simulink model "chap1_4"  (Simulink 3.00)
settings: Solver=ode45  StartTime=0.0  StopTime=5  RelTol=1e-3
libraries: simulink3 x1, simulink_extras x1

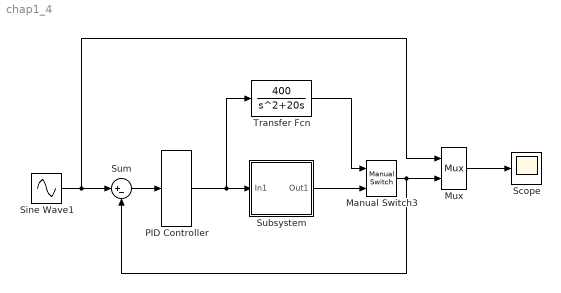
== system chap1_4 ==
  Manual Switch3 : simulink3/Nonlinear/Manual Switch  sw=0  action=0
  Mux : Mux  Inputs=2
      settings: DisplayOption=none
  PID Controller : simulink_extras/Additional Linear/PID Controller  P=10  I=0  D=1
  Scope : Scope
      settings: TimeRange=auto  YMin=-5  YMax=5  SaveToWorkspace=off  SaveName=ScopeData
  Sine Wave1 : Sin  Amplitude=0.50  Frequency=1*2*pi  Phase=0  SampleTime=0
  Subsystem : Subsystem
  Sum : Sum  Inputs=|+-  SaturateOnIntegerOverflow=on
  Transfer Fcn : TransferFcn  Numerator=[400]  Denominator=[1 20 0]
  wires:
  Sum/1 -> PID Controller/1
  Sine Wave1/1 -> Sum/1, Mux/1
  Mux/1 -> Scope/1
  Subsystem/1(Out1) -> Manual Switch3/2
  Transfer Fcn/1 -> Manual Switch3/1
  PID Controller/1 -> Subsystem/1(In1), Transfer Fcn/1
  Manual Switch3/1 -> Mux/2, Sum/2

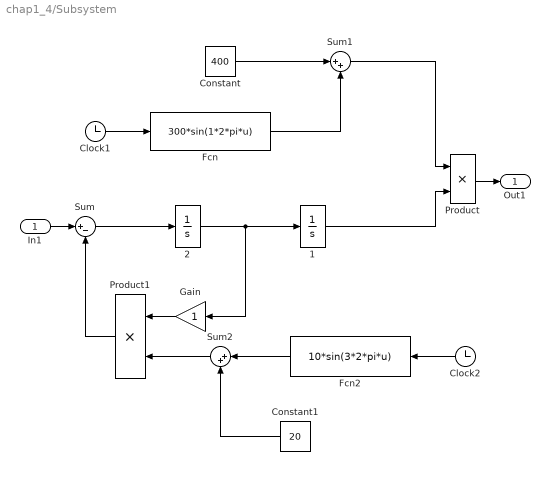
== system chap1_4/Subsystem ==
  In1 : Inport  Port=1  PortWidth=-1  SampleTime=-1  DataType=auto
      settings: SignalType=auto
  " 1" : Integrator  ExternalReset=none  InitialConditionSource=internal  InitialCondition=0  LimitOutput=off  UpperSaturationLimit=inf  LowerSaturationLimit=-inf  ShowSaturationPort=off  ShowStatePort=off  AbsoluteTolerance=auto
  " 2" : Integrator  ExternalReset=none  InitialConditionSource=internal  InitialCondition=0  LimitOutput=off  UpperSaturationLimit=inf  LowerSaturationLimit=-inf  ShowSaturationPort=off  ShowStatePort=off  AbsoluteTolerance=auto
  Clock1 : Clock
  Clock2 : Clock
  Constant : Constant  Value=400
  Constant1 : Constant  Orientation=left  Value=20
  "Fcn " : Fcn  Expr=300*sin(1*2*pi*u)
  Fcn2 : Fcn  Orientation=left  Expr=10*sin(3*2*pi*u)
  Gain : Gain  Orientation=left  Gain=1  SaturateOnIntegerOverflow=on
  Product : Product  Inputs=2  SaturateOnIntegerOverflow=on
  Product1 : Product  Orientation=left  Inputs=2  SaturateOnIntegerOverflow=on
  Sum : Sum  Inputs=|+-  SaturateOnIntegerOverflow=on
  Sum1 : Sum  Inputs=|++  SaturateOnIntegerOverflow=on
  Sum2 : Sum  Orientation=left  Inputs=|++  SaturateOnIntegerOverflow=on
  Out1 : Outport  Port=1
  wires:
  Sum/1 -> " 2"/1
  Clock1/1 -> "Fcn "/1
  " 1"/1 -> Product/2
  " 2"/1 -> " 1"/1, Gain/1
  Clock2/1 -> Fcn2/1
  Gain/1 -> Product1/1
  Product1/1 -> Sum/2
  Product/1 -> Out1/1
  In1/1 -> Sum/1
  "Fcn "/1 -> Sum1/2
  Constant/1 -> Sum1/1
  Sum1/1 -> Product/1
  Fcn2/1 -> Sum2/1
  Sum2/1 -> Product1/2
  Constant1/1 -> Sum2/2
